simulink model "DSF_CANoe_A3"  (R2022b)
settings: configuration reference "CommonModelConfiguration" (kept outside this file)
undefined symbols (not defined in the file or in its folder): OnOff1, PsdNotPsd
libraries: canoelib x127, simulink x44
(part 3 of 3)

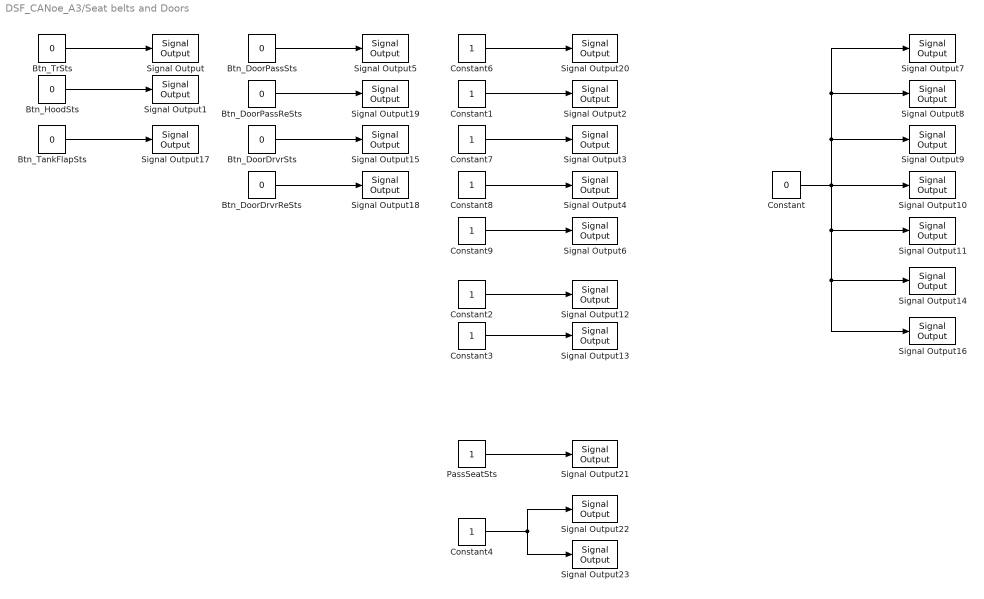
== system DSF_CANoe_A3/Seat belts and Doors ==
  Btn_DoorDrvrReSts : Constant  Value=0
  Btn_DoorDrvrSts : Constant  Value=0
  Btn_DoorPassReSts : Constant  Value=0
  Btn_DoorPassSts : Constant  Value=0
  Btn_HoodSts : Constant  Value=0
  Btn_TankFlapSts : Constant  Value=0
  Btn_TrSts : Constant  Value=0  OutDataTypeStr=uint8
  Constant : Constant  Value=0
  Constant{1..4,6..9} (8 alike) : Constant
  PassSeatSts : Constant
  Signal Output : canoelib/CANoe I//O/Signal Output  dbName=Backbone  nodeName=CEM  msgName=CEMBackBoneSignalIpdu01  sigName=TrSts  rawValue=Default  dataType=Default  dataTypeDB=uint8  hasEncoding=off
      settings: AttributesFormatString=%<sigName>  SourceProductName=Vector CANoe
  Signal Output1 : canoelib/CANoe I//O/Signal Output  dbName=Backbone  nodeName=CEM  msgName=CEMBackBoneSignalIpdu01  sigName=HoodSts  rawValue=Default  dataType=Default  dataTypeDB=uint8  hasEncoding=off
      settings: AttributesFormatString=%<sigName>  SourceProductName=Vector CANoe
  Signal Output10 : canoelib/CANoe I//O/Signal Output  dbName=Backbone  nodeName=SRS  msgName=SRSBackboneSignalIPdu02  sigName=BltLockStAtRowSecMidForBltLockSts  rawValue=Default  dataType=Default  dataTypeDB=boolean  hasEncoding=off
      settings: AttributesFormatString=%<sigName>  SourceProductName=Vector CANoe
  Signal Output11 : canoelib/CANoe I//O/Signal Output  dbName=Backbone  nodeName=SRS  msgName=SRSBackboneSignalIPdu02  sigName=BltLockStAtRowSecRiForBltLockSts  rawValue=Default  dataType=Default  dataTypeDB=boolean  hasEncoding=off
      settings: AttributesFormatString=%<sigName>  SourceProductName=Vector CANoe
  Signal Output12 : canoelib/CANoe I//O/Signal Output  dbName=Backbone  nodeName=SRS  msgName=SRSBackboneSignalIPdu02  sigName=BltLockStAtRowThrdLeForBltLockSt1  rawValue=Default  dataType=Default  dataTypeDB=boolean  hasEncoding=off
      settings: AttributesFormatString=%<sigName>  SourceProductName=Vector CANoe
  Signal Output13 : canoelib/CANoe I//O/Signal Output  dbName=Backbone  nodeName=SRS  msgName=SRSBackboneSignalIPdu02  sigName=BltLockStAtRowThrdRiForBltLockSt1  rawValue=Default  dataType=Default  dataTypeDB=boolean  hasEncoding=off
      settings: AttributesFormatString=%<sigName>  SourceProductName=Vector CANoe
  Signal Output14 : canoelib/CANoe I//O/Signal Output  dbName=Backbone  nodeName=SRS  msgName=SRSBackboneSignalIPdu02  sigName=BltLockStAtRowThrdLeForBltLockSts  rawValue=Default  dataType=Default  dataTypeDB=boolean  hasEncoding=off
      settings: AttributesFormatString=%<sigName>  SourceProductName=Vector CANoe
  Signal Output15 : canoelib/CANoe I//O/Signal Output  dbName=Backbone  nodeName=CEM  msgName=CEMBackBoneSignalIpdu01  sigName=DoorDrvrSts  rawValue=Default  dataType=Default  dataTypeDB=uint8  hasEncoding=off
      settings: AttributesFormatString=%<sigName>  SourceProductName=Vector CANoe
  Signal Output16 : canoelib/CANoe I//O/Signal Output  dbName=Backbone  nodeName=SRS  msgName=SRSBackboneSignalIPdu02  sigName=BltLockStAtRowThrdRiForBltLockSts  rawValue=Default  dataType=Default  dataTypeDB=boolean  hasEncoding=off
      settings: AttributesFormatString=%<sigName>  SourceProductName=Vector CANoe
  Signal Output17 : canoelib/CANoe I//O/Signal Output  dbName=Backbone  nodeName=CEM  msgName=CEMBackBoneSignalIpdu05  sigName=TankFlapSts  rawValue=Default  dataType=Default  dataTypeDB=uint8  hasEncoding=off
      settings: AttributesFormatString=%<sigName>  SourceProductName=Vector CANoe
  Signal Output18 : canoelib/CANoe I//O/Signal Output  dbName=Backbone  nodeName=CEM  msgName=CEMBackBoneSignalIpdu03  sigName=DoorDrvrReSts  rawValue=Default  dataType=Default  dataTypeDB=uint8  hasEncoding=off
      settings: AttributesFormatString=%<sigName>  SourceProductName=Vector CANoe
  Signal Output19 : canoelib/CANoe I//O/Signal Output  dbName=Backbone  nodeName=CEM  msgName=CEMBackBoneSignalIpdu01  sigName=DoorPassReSts  rawValue=Default  dataType=Default  dataTypeDB=uint8  hasEncoding=off
      settings: AttributesFormatString=%<sigName>  SourceProductName=Vector CANoe
  Signal Output2 : canoelib/CANoe I//O/Signal Output  dbName=Backbone  nodeName=SRS  msgName=SRSBackboneSignalIPdu02  sigName=BltLockStAtPassForBltLockSt1  rawValue=Default  dataType=Default  dataTypeDB=boolean  hasEncoding=off
      settings: AttributesFormatString=%<sigName>  SourceProductName=Vector CANoe
  Signal Output20 : canoelib/CANoe I//O/Signal Output  dbName=Backbone  nodeName=SRS  msgName=SRSBackboneSignalIPdu01  sigName=BltLockStAtDrvrForBltLockSt1  rawValue=Default  dataType=Default  dataTypeDB=boolean  hasEncoding=off
      settings: AttributesFormatString=%<sigName>  SourceProductName=Vector CANoe
  Signal Output21 : canoelib/CANoe I//O/Signal Output  dbName=Backbone  nodeName=SRS  msgName=SRSBackboneSignalIPdu03  sigName=PassSeatSts  rawValue=Default  dataType=Default  dataTypeDB=uint8  hasEncoding=off
      settings: AttributesFormatString=%<sigName>  SourceProductName=Vector CANoe
  Signal Output22 : canoelib/CANoe I//O/Signal Output  dbName=Backbone  nodeName=SRS  msgName=SRSBackboneSignalIPdu02  sigName=BltLockStAtRowThrdRiForBltLockEquid  rawValue=Default  dataType=Default  dataTypeDB=boolean  hasEncoding=off
      settings: AttributesFormatString=%<sigName>  SourceProductName=Vector CANoe
  Signal Output23 : canoelib/CANoe I//O/Signal Output  dbName=Backbone  nodeName=SRS  msgName=SRSBackboneSignalIPdu02  sigName=BltLockStAtRowThrdLeForBltLockEquid  rawValue=Default  dataType=Default  dataTypeDB=boolean  hasEncoding=off
      settings: AttributesFormatString=%<sigName>  SourceProductName=Vector CANoe
  Signal Output3 : canoelib/CANoe I//O/Signal Output  dbName=Backbone  nodeName=SRS  msgName=SRSBackboneSignalIPdu02  sigName=BltLockStAtRowSecLeForBltLockSt1  rawValue=Default  dataType=Default  dataTypeDB=boolean  hasEncoding=off
      settings: AttributesFormatString=%<sigName>  SourceProductName=Vector CANoe
  Signal Output4 : canoelib/CANoe I//O/Signal Output  dbName=Backbone  nodeName=SRS  msgName=SRSBackboneSignalIPdu02  sigName=BltLockStAtRowSecMidForBltLockSt1  rawValue=Default  dataType=Default  dataTypeDB=boolean  hasEncoding=off
      settings: AttributesFormatString=%<sigName>  SourceProductName=Vector CANoe
  Signal Output5 : canoelib/CANoe I//O/Signal Output  dbName=Backbone  nodeName=CEM  msgName=CEMBackBoneSignalIpdu01  sigName=DoorPassSts  rawValue=Default  dataType=Default  dataTypeDB=uint8  hasEncoding=off
      settings: AttributesFormatString=%<sigName>  SourceProductName=Vector CANoe
  Signal Output6 : canoelib/CANoe I//O/Signal Output  dbName=Backbone  nodeName=SRS  msgName=SRSBackboneSignalIPdu02  sigName=BltLockStAtRowSecRiForBltLockSt1  rawValue=Default  dataType=Default  dataTypeDB=boolean  hasEncoding=off
      settings: AttributesFormatString=%<sigName>  SourceProductName=Vector CANoe
  Signal Output7 : canoelib/CANoe I//O/Signal Output  dbName=Backbone  nodeName=SRS  msgName=SRSBackboneSignalIPdu01  sigName=BltLockStAtDrvrForDevErrSts2  rawValue=Default  dataType=Default  dataTypeDB=boolean  hasEncoding=off
      settings: AttributesFormatString=%<sigName>  SourceProductName=Vector CANoe
  Signal Output8 : canoelib/CANoe I//O/Signal Output  dbName=Backbone  nodeName=SRS  msgName=SRSBackboneSignalIPdu02  sigName=BltLockStAtPassForBltLockSts  rawValue=Default  dataType=Default  dataTypeDB=boolean  hasEncoding=off
      settings: AttributesFormatString=%<sigName>  SourceProductName=Vector CANoe
  Signal Output9 : canoelib/CANoe I//O/Signal Output  dbName=Backbone  nodeName=SRS  msgName=SRSBackboneSignalIPdu02  sigName=BltLockStAtRowSecLeForBltLockSts  rawValue=Default  dataType=Default  dataTypeDB=boolean  hasEncoding=off
      settings: AttributesFormatString=%<sigName>  SourceProductName=Vector CANoe
  wires:
  Btn_DoorDrvrReSts/1 -> Signal Output18/1
  Btn_DoorDrvrSts/1 -> Signal Output15/1
  Btn_DoorPassReSts/1 -> Signal Output19/1
  Btn_DoorPassSts/1 -> Signal Output5/1
  Constant6/1 -> Signal Output20/1
  Btn_HoodSts/1 -> Signal Output1/1
  Btn_TrSts/1 -> Signal Output/1
  Constant9/1 -> Signal Output6/1
  Constant7/1 -> Signal Output3/1
  Constant1/1 -> Signal Output2/1
  Constant8/1 -> Signal Output4/1
  Constant/1 -> Signal Output7/1, Signal Output8/1, Signal Output9/1, Signal Output16/1, Signal Output14/1, Signal Output11/1, Signal Output10/1
  Constant3/1 -> Signal Output13/1
  Constant2/1 -> Signal Output12/1
  Btn_TankFlapSts/1 -> Signal Output17/1
  PassSeatSts/1 -> Signal Output21/1
  Constant4/1 -> Signal Output22/1, Signal Output23/1

== system DSF_CANoe_A3/Speed limit model ==
  SpdLim_up : Inport
  SpdLim_down : Inport  Port=2
  SpdLimFirst : Inport  Port=3
  SpdLimSec : Inport  Port=4
  AccSts : Inport  Port=5
  CC_Sts : Inport  Port=6
  SL_Sts : Inport  Port=7
  SetSpeed : Inport  Port=8
  SLA/SpdLim : Stateflow chart  TreatAsAtomicUnit=on
      settings: PortSchema="{\"entries\":[{\"content\":{\"sides\":[{\"content\":{\"connectorIds\":[\"In1\",\"In2\",\"In3\",\"In4\",\"In5\",\"In6\",\"In7\",\"In8\"]},\"type\":\"ConnectorPlacement.EquallySpacedRectSide\",\"uuid\":\"50a9cfe1-14d0-4131-bd43-42b01cfb3bc1\"},{\"content\":{\"connectorIds\":[\"Out2\",\"Out1\",\"Out3\",\"Out4\"],\"side\":\"RIGHT\"},\"type\":\"ConnectorPlacement.EquallySpacedRectSide\",\"uuid\":\"e893b316-2b3e-4fbb-8898-380048607deb\"},{\"content\":{\"connectorIds\":[],\"side\":\"TOP\"},\"type\":\"ConnectorPlacement.EquallySpacedRectSide\",\"uuid\":\"15802024-6082-4699-9c20-01ccd97957b8\"}]},\"type\":\"ConnectorPlacement.EquallySpacedConnector\",\"uuid\":\"0bbff380-7a2f-4c63-8641-ffef81eb902e\"}],\"packageUris\":[\"http://schema.mathworks.com/mf0/Connector/R2020b\"],\"version\":\"1.0\"}"
  SET_SpdLimFirst : Outport
  SET_SpdLimSec : Outport  Port=2
  SET_SetSpdSelnForAutDrv : Outport  Port=3
  SET_SpdLimAdpvActv : Outport  Port=4
  wires:
  SLA/SpdLim/2(SET_SpdLimFirst) -> SET_SpdLimFirst/1
  SLA/SpdLim/1(SET_SpdLimSec) -> SET_SpdLimSec/1
  SpdLim_down/1 -> SLA/SpdLim/2(PushDown)
  SpdLim_up/1 -> SLA/SpdLim/1(PushUp)
  SpdLimFirst/1 -> SLA/SpdLim/3(SpdLimFirst)
  SpdLimSec/1 -> SLA/SpdLim/4(SpdLimSec)
  SLA/SpdLim/3(SET_SetSpdSelnForAutDrv) -> SET_SetSpdSelnForAutDrv/1
  SLA/SpdLim/4(SET_SpdLimAdpvActv) -> SET_SpdLimAdpvActv/1
  AccSts/1 -> SLA/SpdLim/5(AccSts)
  CC_Sts/1 -> SLA/SpdLim/6(CC_Sts)
  SL_Sts/1 -> SLA/SpdLim/7(SL_Sts)
  SetSpeed/1 -> SLA/SpdLim/8(SetSpeed)

== system DSF_CANoe_A3/Timegap ==
  Constant25 : Constant  OutDataTypeStr=uint8
  Constant5 : Constant  OutDataTypeStr=uint8
  Display50 : Display
  Display52 : Display
  Signal Input10 : canoelib/CANoe I//O/Signal Input  dbName=Backbone  nodeName=DIM  msgName=DIMBackBoneSignalIPdu05  sigName=TiGapAdpvSts  editSampleTime=0  rawValue=Default  dataType=Default  dataTypeDB=boolean  hasEncoding=off
      settings: AttributesFormatString=%<sigName>  SourceProductName=Vector CANoe
  Signal Input9 : canoelib/CANoe I//O/Signal Input  dbName=Backbone  nodeName=DIM  msgName=DIMBackBoneSignalIPdu04  sigName=TiGapSts  editSampleTime=0  rawValue=Default  dataType=Default  dataTypeDB=uint8  hasEncoding=on
      settings: AttributesFormatString=%<sigName>  SourceProductName=Vector CANoe
  Signal Output48 : canoelib/CANoe I//O/Signal Output  dbName=Backbone  nodeName=ASDM  msgName=ASDMBackBoneSignalIPdu06  sigName=TiGapAdpv  rawValue=Default  dataType=Default  dataTypeDB=uint8  hasEncoding=on
      settings: AttributesFormatString=%<sigName>  SourceProductName=Vector CANoe
  Signal Output49 : canoelib/CANoe I//O/Signal Output  dbName=Backbone  nodeName=IHU  msgName=IHUBackBoneSignalIPdu05  sigName=TiGapLimdSts  rawValue=Default  dataType=Default  dataTypeDB=uint8  hasEncoding=on
      settings: AttributesFormatString=%<sigName>  SourceProductName=Vector CANoe
  wires:
  Signal Input9/1 -> Display50/1
  Constant5/1 -> Signal Output49/1
  Constant25/1 -> Signal Output48/1
  Signal Input10/1 -> Display52/1

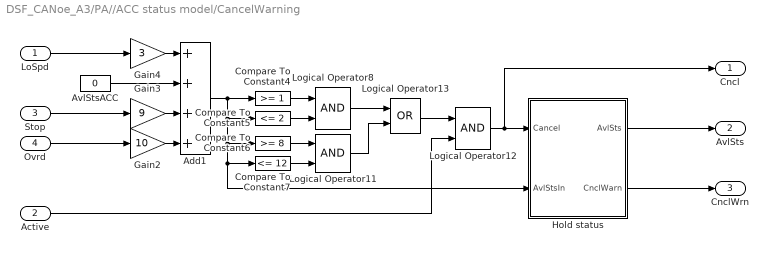
== system DSF_CANoe_A3/PA//ACC status model/CancelWarning ==
  LoSpd : Inport
  Active : Inport  Port=2
  Stop : Inport  Port=3
  Ovrd : Inport  Port=4
  Add1 : Sum  Inputs=++++
  AvlStsACC : Constant  Value=0
  Compare To Constant4 : simulink/Logic and Bit Operations/Compare To Constant  relop=>=  const=1  OutDataTypeStr=boolean
  Compare To Constant5 : simulink/Logic and Bit Operations/Compare To Constant  relop=<=  const=2  OutDataTypeStr=boolean
  Compare To Constant6 : simulink/Logic and Bit Operations/Compare To Constant  relop=>=  const=8  OutDataTypeStr=boolean
  Compare To Constant7 : simulink/Logic and Bit Operations/Compare To Constant  relop=<=  const=12  OutDataTypeStr=boolean
  Gain2 : Gain  Gain=10  OutDataTypeStr=double
  Gain3 : Gain  Gain=9  OutDataTypeStr=double
  Gain4 : Gain  Gain=3  OutDataTypeStr=double
  Hold status : Stateflow chart  TreatAsAtomicUnit=on
  Logical Operator11 : Logic  AllPortsSameDT=off  OutDataTypeStr=boolean
  Logical Operator12 : Logic  AllPortsSameDT=off  OutDataTypeStr=boolean
  Logical Operator13 : Logic  Operator=OR  AllPortsSameDT=off  OutDataTypeStr=boolean
  Logical Operator8 : Logic  AllPortsSameDT=off  OutDataTypeStr=boolean
  Cncl : Outport
  AvlSts : Outport  Port=2
  CnclWrn : Outport  Port=3
  wires:
  LoSpd/1 -> Gain4/1
  Logical Operator8/1 -> Logical Operator13/1
  Logical Operator11/1 -> Logical Operator13/2
  Compare To Constant4/1 -> Logical Operator8/1
  Compare To Constant5/1 -> Logical Operator8/2
  Compare To Constant6/1 -> Logical Operator11/1
  Compare To Constant7/1 -> Logical Operator11/2
  Logical Operator13/1 -> Logical Operator12/1
  Active/1 -> Logical Operator12/2
  Logical Operator12/1 -> Cncl/1, Hold status/1(Cancel)
  Gain3/1 -> Add1/3
  AvlStsACC/1 -> Add1/2
  Gain2/1 -> Add1/4
  Gain4/1 -> Add1/1
  Ovrd/1 -> Gain2/1
  Stop/1 -> Gain3/1
  Add1/1 -> Hold status/2(AvlStsIn), Compare To Constant7/1, Compare To Constant6/1, Compare To Constant5/1, Compare To Constant4/1
  Hold status/1(AvlSts) -> AvlSts/1
  Hold status/2(CnclWarn) -> CnclWrn/1

== stateflow chart DSF_CANoe_A3/ISA model/Chart1 ==
  state WARNING_ON
    en, du: SET_SpdLimAudWarnReq = 1;
  state WARNING_OFF
    en, du: SET_SpdLimAudWarnReq = 0;
  (default) -> WARNING_OFF
  WARNING_OFF -> WARNING_ON : %Speed limit exceeded
      | [hasChangedTo(SpdLimitExcd, true)]
  WARNING_ON -> WARNING_OFF : %Request times out
      | after(3, sec)
  data: SpdLimitExcd input; SET_SpdLimAudWarnReq output

== stateflow chart DSF_CANoe_A3/Speed limit model/SLA//SpdLim ==
  state NEW_SPEED_LIMIT
    entry:
    SET_SetSpdSelnForAutDrv = 1;
    SET_SpdLimAdpvActv = 0;
  state SHOW
  state WAIT1
  state ACTIVATE_SLA
    entry:
    SET_SpdLimAdpvActv = 1;
  state WAIT2
  (default) -> NEW_SPEED_LIMIT : {SET_SpdLimFirst = SpdLimFirst;
      | SET_SpdLimSec = SpdLimSec;}
  (junction 75) -> SHOW [order 2]
  SHOW -> WAIT1 : [after(2, sec)]
      | {SET_SpdLimFirst = SET_SpdLimSec;
      | SET_SpdLimSec = 0;}
  NEW_SPEED_LIMIT -> (junction 75) [order 2] : [PushUp==PsdNotPsd.PsdNotPsd_Psd &&...
      | SET_SpdLimFirst <= 150]
      | {SET_SpdLimSec = SET_SpdLimFirst + 10;}
  (junction 75) -> SHOW [order 1] : [SET_SpdLimSec==150]
      | {SET_SpdLimSec = 254;}
  WAIT1 -> ACTIVATE_SLA : [after(0.1, sec)]
  (junction 83) -> SHOW [order 1] : [SL_Sts==3]
  (junction 80) -> (junction 83) [order 2]
  NEW_SPEED_LIMIT -> (junction 80) [order 1] : [PushDown==PsdNotPsd.PsdNotPsd_Psd &&...
      | SET_SpdLimFirst >= 20]...
      | {SET_SpdLimSec = SET_SpdLimFirst - 10;}
  (junction 80) -> (junction 83) [order 1] : [SET_SpdLimSec>130]
      | {SET_SpdLimSec = 130;}
  (junction 83) -> WAIT2 [order 2] : {SET_SetSpdSelnForAutDrv = 2;}
  WAIT2 -> ACTIVATE_SLA : [after(0.1, sec)]
  NEW_SPEED_LIMIT -> ACTIVATE_SLA [order 3] : [(hasChangedTo(AccSts, 5) || hasChangedTo(CC_Sts, 3) ||...
      | hasChangedTo(SL_Sts, 3)) && SetSpeed<SpdLimFirst]
      | {SET_SetSpdSelnForAutDrv = 1;}
  (junction 90) -> NEW_SPEED_LIMIT [order 1] : [SET_SpdLimSec~=0]
      | {SET_SpdLimFirst = SET_SpdLimSec; SET_SpdLimSec = 0;}
  ACTIVATE_SLA -> (junction 90) : [after(2, sec)]
  (junction 90) -> NEW_SPEED_LIMIT [order 2]
  data: SET_SpdLimSec output; SET_SpdLimFirst output; PushUp input; PushDown input; SpdLimFirst input; SpdLimSec input; SET_SetSpdSelnForAutDrv output; SET_SpdLimAdpvActv output; AccSts input; CC_Sts input; SL_Sts input; SetSpeed input

== stateflow chart DSF_CANoe_A3/LCA model/Hold status ==
  state HOLD_AVAILABILITY
    entry:
    LC_sts = StsIn;
    AvlSts = AvlStsIn;
  state CURRENT_AVAILABILITY
    en, du:
    LC_sts = StsIn;
    AvlSts = AvlStsIn;
  (default) -> CURRENT_AVAILABILITY
  CURRENT_AVAILABILITY -> HOLD_AVAILABILITY : %Cancel condition
      | [hasChangedTo(Cancel, true)]
  HOLD_AVAILABILITY -> CURRENT_AVAILABILITY : %Hold timeout
      | [after(2, sec)]
  data: StsIn input; AvlSts output; Cancel input; LC_sts output; AvlStsIn input

== stateflow chart DSF_CANoe_A3/LCA model/LaneChgLe ==
  state TURNING_OFF
    en, du:
    TurnPeriod = false;
    Cancel = false;
  state TURNING_ON
    en, du:
    TurnPeriod = true;
  state TURNING_CANCEL
    en, du:
    TurnPeriod = false;
    Cancel = true;
  (default) -> TURNING_OFF
  TURNING_OFF -> TURNING_ON : %Indicator on
      | [hasChangedTo(TurnSignal, 1) && Psbl]
  TURNING_ON -> TURNING_OFF [order 1] : %Lane changed cancelled or finished
      | [hasChangedTo(Cncl, 1) || after(15, sec)]
  TURNING_CANCEL -> TURNING_OFF : [after(3, sec)]
  TURNING_ON -> TURNING_CANCEL [order 2] : %Cancelled by driver, indicator off
      | [hasChangedTo(TurnSignal, 0)]
  data: TurnSignal input; TurnPeriod output; Cncl input; Psbl input; Cancel output

== stateflow chart DSF_CANoe_A3/LCA model/LaneChgRi ==
  state TURNING_OFF
    en, du:
    TurnPeriod = false;
    Cancel = false;
  state TURNING_ON
    en, du:
    TurnPeriod = true;
  state TURNING_CANCEL
    en, du:
    TurnPeriod = false;
    Cancel = true;
  (default) -> TURNING_OFF
  TURNING_OFF -> TURNING_ON : %Indicator on
      | [hasChangedTo(TurnSignal, 1) && Psbl]
  TURNING_ON -> TURNING_OFF [order 1] : %Lane changed cancelled or finished
      | [hasChangedTo(Cncl, 1) || after(15, sec)]
  TURNING_CANCEL -> TURNING_OFF : [after(3, sec)]
  TURNING_ON -> TURNING_CANCEL [order 2] : %Cancelled by driver, indicator off
      | [hasChangedTo(TurnSignal, 0)]
  data: TurnSignal input; TurnPeriod output; Cncl input; Psbl input; Cancel output

== stateflow chart DSF_CANoe_A3/PA//ACC status model/Override timeout ==
  state TIMER_ON
  state TIMER_OFF
    en, du: Timeout = false;
  state TIMEOUT
    en, du: Timeout = true;
  (default) -> TIMER_OFF
  TIMER_OFF -> TIMER_ON : %Timer on
      | [hasChangedTo(Set, true)]
  TIMER_ON -> TIMER_OFF [order 2] : %Timer off
      | [hasChangedTo(Set, false)]
  TIMEOUT -> TIMER_OFF : %Reset timer
      | [after(3, sec)]
  TIMER_ON -> TIMEOUT [order 1] : %Timeout reached
      | [after(Time, sec)]
  data: Set input; Timeout output; Time input

== stateflow chart DSF_CANoe_A3/HOW model/ESA//deactivate timer ==
  state TIMER_ON
  state TIMER_OFF
    en, du: Timeout = false;
  state TIMEOUT
    en, du: Timeout = true;
  (default) -> TIMER_OFF
  TIMER_OFF -> TIMER_ON : %Timer on
      | [hasChangedTo(Set, true)]
  TIMER_ON -> TIMER_OFF [order 2] : %Timer off
      | [hasChangedTo(Set, false)]
  TIMER_ON -> TIMEOUT [order 1] : %Timeout reached
      | [after(Time, sec)]
  (junction 19) -> TIMER_OFF : [after(3, sec)]
  TIMEOUT -> (junction 19) : %Reset timer
      | [hasChangedTo(Set, false) ||...
      | hasChangedTo(PA_act, false)]
  data: Set input; Timeout output; Time input; PA_act input

== stateflow chart DSF_CANoe_A3/HOW model/Level 1 timer ==
  state TIMER_ON
  state TIMER_OFF
    en, du: Timeout = false;
  state TIMEOUT
    en, du: Timeout = true;
  (default) -> TIMER_OFF
  TIMER_OFF -> TIMER_ON : %Timer on
      | [hasChangedTo(Set, true)]
  TIMER_ON -> TIMER_OFF [order 2] : %Timer off
      | [hasChangedTo(Set, false)]
  TIMEOUT -> TIMER_OFF : %Reset timer
      | [hasChangedTo(Set, false)]
  TIMER_ON -> TIMEOUT [order 1] : %Timeout reached
      | [after(Time, sec)]
  data: Set input; Timeout output; Time input

== stateflow chart DSF_CANoe_A3/HOW model/Level 2 timer ==
  state TIMER_ON
  state TIMER_OFF
    en, du: Timeout = false;
  state TIMEOUT
    en, du: Timeout = true;
  (default) -> TIMER_OFF
  TIMER_OFF -> TIMER_ON : %Timer on
      | [hasChangedTo(Set, true)]
  TIMER_ON -> TIMER_OFF [order 2] : %Timer off
      | [hasChangedTo(Set, false)]
  TIMEOUT -> TIMER_OFF : %Reset timer
      | [hasChangedTo(Set, false)]
  TIMER_ON -> TIMEOUT [order 1] : %Timeout reached
      | [after(Time, sec)]
  data: Set input; Timeout output; Time input

== stateflow chart DSF_CANoe_A3/PA//ACC status model/CancelWarning/Hold status ==
  state HOLD_AVAILABILITY
    entry:
    CnclWarn = 2;
    AvlSts = AvlStsIn;
  state CURRENT_AVAILABILITY
    en, du:
    CnclWarn = 1;
    AvlSts = AvlStsIn;
  (default) -> CURRENT_AVAILABILITY
  CURRENT_AVAILABILITY -> HOLD_AVAILABILITY : %Cancel condition
      | [hasChangedTo(Cancel, true)]
  HOLD_AVAILABILITY -> CURRENT_AVAILABILITY : %Hold timeout
      | [after(2, sec)]
  data: AvlSts output; Cancel input; CnclWarn output; AvlStsIn input

== stateflow chart DSF_CANoe_A3/CC model/CrsCtrlState ==
  state CC_OFF
    en, du: State = 1;
  state CC_ACTIVE
    en, du: State = 3;
  state CC_STBY
    en, du: State = 2;
  (default) -> CC_OFF
  CC_OFF -> CC_STBY : %CC selected
      | [CrsCtrlFctSeld==2]
  CC_STBY -> CC_OFF [order 2] : %CC not selected
      | [CrsCtrlFctSeld~=2]
  CC_STBY -> CC_ACTIVE [order 1] : %Activate CC
      | [hasChangedTo(Activate, true)]
  CC_ACTIVE -> CC_STBY : %CC standby
      | [hasChangedTo(Deactivate, true)]
  data: CrsCtrlFctSeld input; Activate input; State output; Deactivate input

== stateflow chart DSF_CANoe_A3/PA//ACC status model/ACC_State ==
  state ACC_OFF
    en, du: State = 1;
  state ACC_ACTIVE
    en, du: State = 5;
  state ACC_STBY
    en, du: State = 2;
  state STOPPED
  state ACC_STOP
    en, du: State = 3;
  (default) -> ACC_OFF
  ACC_OFF -> ACC_STBY : %ACC selected
      | [CrsCtrlFctSeld==3]
  ACC_STBY -> ACC_OFF [order 2] : %ACC not selected
      | [CrsCtrlFctSeld~=3]
  ACC_STBY -> ACC_ACTIVE [order 1] : %Activate ACC
      | [hasChangedTo(Activate, true)]
  ACC_ACTIVE -> ACC_STBY [order 1] : %ACC standby
      | [hasChangedTo(Deactivate, true)]
  ACC_STOP -> ACC_STBY [order 2] : [hasChangedTo(Deactivate, true)]
  ACC_ACTIVE -> STOPPED [order 2] : [SpdTar==0]
  STOPPED -> ACC_ACTIVE [order 2] : [SpdTar~=0]
  ACC_STOP -> ACC_ACTIVE [order 1] : [hasChangedTo(Activate, true)]
  STOPPED -> ACC_STOP [order 1] : [after(3, sec)]
  data: SpdTar input; CrsCtrlFctSeld input; Activate input; State output; Deactivate input

== stateflow chart DSF_CANoe_A3/SL model/SL_State ==
  state SL_OFF
    en, du: State = 1;
  state SL_STBY
    en, du: State = 2;
  state SL_ACTIVE
    en, du: State = 3;
  state SL_OVERRIDDEN
    en, du: State = 4;
  (default) -> SL_OFF
  SL_OFF -> SL_STBY : %SL selected
      | [CrsCtrlFctSeld==1]
  SL_STBY -> SL_OFF [order 2] : %SL not selected
      | [CrsCtrlFctSeld~=1]
  SL_STBY -> SL_ACTIVE [order 1] : %Activate SL
      | [hasChangedTo(Activate, true)]
  SL_ACTIVE -> SL_STBY [order 1] : %SL standby
      | [hasChangedTo(Deactivate, true)]
  SL_OVERRIDDEN -> SL_STBY [order 2] : [hasChangedTo(Deactivate, true)]
  SL_ACTIVE -> SL_OVERRIDDEN [order 2] : [CrsCtrlOvrdn==1]
  SL_OVERRIDDEN -> SL_ACTIVE [order 1] : [CrsCtrlOvrdn==0]
  data: CrsCtrlFctSeld input; Activate input; State output; Deactivate input; CrsCtrlOvrdn input

== stateflow chart DSF_CANoe_A3/PA//ACC status model/Misuse ==
  state STEER_OFF
    en, du: NoSteer = true;
  state STEER_ON
    en, du: NoSteer = false;
  (default) -> STEER_ON
  STEER_ON -> STEER_OFF : %Hands off wheel for too long
      | [hasChangedTo(EmgStop, true)]
  data: EmgStop input; NoSteer output

== stateflow chart DSF_CANoe_A3/PA//ACC status model/Stop timeout ==
  state TIMEOUT_OFF
    en, du: Timeout = false;
  state TIMER_ON
  state TIMEOUT_ON
    en, du: Timeout = true;
  (default) -> TIMEOUT_OFF
  TIMEOUT_OFF -> TIMER_ON : %Stop mode initiated
      | [hasChangedTo(State, 3)]
  TIMER_ON -> TIMEOUT_OFF [order 1] : %Activated, reset
      | [hasChangedTo(State, 5)]
  TIMER_ON -> TIMEOUT_ON [order 2] : %Timeout reached
      | [after(Time, sec)]
  TIMEOUT_ON -> TIMEOUT_OFF : %Reset timer
      | [after(1, sec)]
  data: State input; Timeout output; Time input

== stateflow chart DSF_CANoe_A3/PA//ACC status model/PA_State ==
  state PA_STBY
    en, du: State = 0;
  state PA_ACTIVE
    en, du: State = 0;
  state STEER_ASSIST_ACTIVE
    en, du: State = 1;
  (default) -> PA_STBY
  PA_STBY -> PA_ACTIVE : %Activate steer assist
      | [hasChangedTo(Activate, 1)]
  PA_ACTIVE -> PA_STBY [order 2] : %Deactivate steer assist
      | [hasChangedTo(Deactivate, 1)]
  STEER_ASSIST_ACTIVE -> PA_STBY [order 2] : %Deactivate steer assist
      | [hasChangedTo(Deactivate, 1)]
  PA_ACTIVE -> STEER_ASSIST_ACTIVE [order 1] : % Activate steering if available
      | [Unavailable==0]
  STEER_ASSIST_ACTIVE -> PA_ACTIVE [order 1] : % Deactivate steering if unavailable
      | [Unavailable==1]
  data: Activate input; State output; Deactivate input; Unavailable input

== matlab function DSF_CANoe_A3/ISA model/MATLAB Function ==
  data: SpdLimAudWarnActvReq input; SpdLimAudWarnSts output
function SpdLimAudWarnSts = SetSpdLimAudWarnSts(SpdLimAudWarnActvReq)

% Toggle SpdLimAudWarnSts on each rising edge of SpdLimAudWarnActvReq

persistent prev_SpdLimAudWarnActvReq state

% Initialize persistent variables as logical
if isempty(prev_SpdLimAudWarnActvReq)
    prev_SpdLimAudWarnActvReq = false;
end

if isempty(state)
    state = false;
end

% Ensure input is logical
SpdLimAudWarnActvReq = logical(SpdLimAudWarnActvReq);

% Detect rising edge
rising_edge = SpdLimAudWarnActvReq && ~prev_SpdLimAudWarnActvReq;

% Toggle state on rising edge
if rising_edge
    state = ~state;
end

% Output latched state
SpdLimAudWarnSts = state;

% Store previous input
prev_SpdLimAudWarnActvReq = SpdLimAudWarnActvReq;

end

== stateflow chart DSF_CANoe_A3/SCF/SCF_SpdCtrlFctStst ==
  (default) -> (junction 68)
  (junction 68) -> (junction 70) [order 1] : [SCF_Status == 1]
  (junction 70) -> (junction 67) [order 1] : [GetAccSts == AccSts1.AccSts1_Actv]
      | {SetSpdCtrlFctSts = 1}
  (junction 68) -> (junction 66) [order 2] : {SetSpdCtrlFctSts = 0}
  (junction 70) -> (junction 71) [order 2]
  (junction 67) -> (junction 69)
  (junction 71) -> (junction 69) : [(GetAccSts == AccSts1.AccSts1_Off) || (GetAccSts == AccSts1.AccSts1_Stb) ]
      | {SetSpdCtrlFctSts = 4}
  (junction 69) -> (junction 60)
  (junction 60) -> (junction 66)
  (junction 66) -> (junction 56)
  data: SCF_Status input; GetAccSts input; SetSpdCtrlFctSts output
